simulink model "test_xeng_2"  (Simulink 7.0)
settings: Solver=ode45  StartTime=0.0  StopTime=200000  RelTol=1e-3
libraries: xbsIndex_r4 x1501, xbsReplacements_r4 x144, casper_library x23, xps_library x2, simulink x1
(part 2 of 16)

== system test_xeng_2/Subsystem/inj_vector1 ==
  In1 : Inport  OutDataType=sfix(16)  OutScaling=2^0
  Product : Product  OutDataType=sfix(16)  OutScaling=2^0  RndMeth=Zero
  err_clear_sim1 : Constant  Value=2^bit_pos  OutDataType=sfix(16)  OutScaling=2^0
  Out1 : Outport  OutDataType=sfix(16)  OutScaling=2^0
  wires:
  err_clear_sim1/1 -> Product/2
  In1/1 -> Product/1
  Product/1 -> Out1/1

== system test_xeng_2/Subsystem/new_acc2 ==
  In1 : Inport  OutDataType=sfix(16)  OutScaling=2^0
  Product : Product  OutDataType=sfix(16)  OutScaling=2^0  RndMeth=Zero
  err_clear_sim1 : Constant  Value=2^bit_pos  OutDataType=sfix(16)  OutScaling=2^0
  Out1 : Outport  OutDataType=sfix(16)  OutScaling=2^0
  wires:
  err_clear_sim1/1 -> Product/2
  In1/1 -> Product/1
  Product/1 -> Out1/1

== system test_xeng_2/Subsystem/run1 ==
  In1 : Inport  OutDataType=sfix(16)  OutScaling=2^0
  Product : Product  OutDataType=sfix(16)  OutScaling=2^0  RndMeth=Zero
  err_clear_sim1 : Constant  Value=2^bit_pos  OutDataType=sfix(16)  OutScaling=2^0
  Out1 : Outport  OutDataType=sfix(16)  OutScaling=2^0
  wires:
  err_clear_sim1/1 -> Product/2
  In1/1 -> Product/1
  Product/1 -> Out1/1

== system test_xeng_2/Subsystem/valid_sel1 ==
  In1 : Inport  OutDataType=sfix(16)  OutScaling=2^0
  Product : Product  OutDataType=sfix(16)  OutScaling=2^0  RndMeth=Zero
  err_clear_sim1 : Constant  Value=2^bit_pos  OutDataType=sfix(16)  OutScaling=2^0
  Out1 : Outport  OutDataType=sfix(16)  OutScaling=2^0
  wires:
  err_clear_sim1/1 -> Product/2
  In1/1 -> Product/1
  Product/1 -> Out1/1

== system test_xeng_2/pkt_reord0/deflagger ==
  din : Inport  OutDataType=sfix(16)  OutScaling=2^0
  Slice1 : xbsIndex_r4/Slice  nbits=16  boolean_output=off  mode=Lower Bit Location + Width  bit1=0  base1=MSB of Input  bit0=0  base0=LSB of Input  dbl_ovrd=off  block_type=slice
      settings: infoedit="Extracts a given range of bits from each input sample and presents it at the output.  The output type is ordinarily unsigned with binary point at zero, but can be Boolean when the slice is one bit wide.<P><P>Hardware notes: In hardware this block costs nothing."  block_version=10.1.3
  Slice2 : xbsIndex_r4/Slice  nbits=1  boolean_output=off  mode=Upper Bit Location + Width  bit1=-1  base1=MSB of Input  bit0=0  base0=LSB of Input  dbl_ovrd=off  block_type=slice
      settings: infoedit="Extracts a given range of bits from each input sample and presents it at the output.  The output type is ordinarily unsigned with binary point at zero, but can be Boolean when the slice is one bit wide.<P><P>Hardware notes: In hardware this block costs nothing."  block_version=10.1.3
  Slice3 : xbsIndex_r4/Slice  nbits=1  boolean_output=off  mode=Upper Bit Location + Width  bit1=0  base1=MSB of Input  bit0=0  base0=LSB of Input  dbl_ovrd=off  block_type=slice
      settings: infoedit="Extracts a given range of bits from each input sample and presents it at the output.  The output type is ordinarily unsigned with binary point at zero, but can be Boolean when the slice is one bit wide.<P><P>Hardware notes: In hardware this block costs nothing."  block_version=10.1.3
  dout : Outport  OutDataType=sfix(16)  OutScaling=2^0
  flag : Outport  Port=2  OutDataType=sfix(16)  OutScaling=2^0
  rcvd : Outport  Port=3  OutDataType=sfix(16)  OutScaling=2^0
  wires:
  Slice1/1 -> dout/1
  Slice3/1 -> rcvd/1
  Slice2/1 -> flag/1
  din/1 -> Slice3/1, Slice2/1, Slice1/1

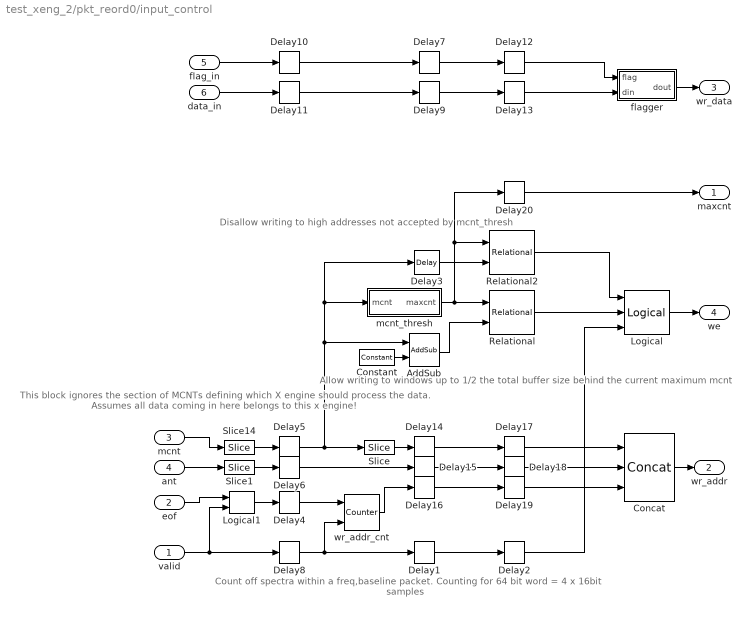
== system test_xeng_2/pkt_reord0/input_control ==
  note: Allow writing to windows
      | up to 1/2 the total buffer size
      |  behind the current maximum mcnt
  note: Count off spectra
      | within a freq,baseline
      | packet.  Counting for
      | 64 bit word = 4 x 16bit samples
  note: Disallow writing to high addresses
      | not accepted by mcnt_thresh
  note: This block ignores the section of
      | MCNTs defining which X engine
      | should process the data.
      | Assumes all data coming in here
      | belongs to this x engine!
  valid : Inport  OutDataType=sfix(16)  OutScaling=2^0
  eof : Inport  Port=2  OutDataType=sfix(16)  OutScaling=2^0
  mcnt : Inport  Port=3  OutDataType=sfix(16)  OutScaling=2^0
  ant : Inport  Port=4  OutDataType=sfix(16)  OutScaling=2^0
  flag_in : Inport  Port=5  OutDataType=sfix(16)  OutScaling=2^0
  data_in : Inport  Port=6  OutDataType=sfix(16)  OutScaling=2^0
  AddSub : xbsIndex_r4/AddSub  mode=Addition  use_carryin=off  use_carryout=off  en=off  latency=2  precision=User Defined  arith_type=Unsigned  n_bits=48 - ant_bits  bin_pt=0  quantization=Truncate  overflow=Wrap  dbl_ovrd=off  use_behavioral_HDL=on  pipelined=off  use_rpm=on  hw_selection=Fabric  block_type=addsub
      settings: xl_area=[0, 0, 0, 0, 0, 0, 0]  block_version=10.1.3
  Concat : xbsIndex_r4/Concat  num_inputs=3  dbl_ovrd=off  block_type=concat
      settings: block_version=10.1.3
  Constant : xbsIndex_r4/Constant  arith_type=Unsigned  const=2^(window_bits - 1)  n_bits=48 - ant_bits  bin_pt=0  explicit_period=on  period=1  equ=P=C  opselect=C  inp2=PCIN>>17  opr=+  inp1=P  carry=CIN  dbl_ovrd=off  block_type=constant
  Delay{1,7,9,14..16} (6 alike) : xbsIndex_r4/Delay  en=off  latency=2  dbl_ovrd=off  reg_retiming=on  block_type=delay
      settings: xl_area=[0, 0, 0, 0, 0, 0, 0]
  Delay{2,4..6,8,10..13,17..20} (13 alike) : xbsIndex_r4/Delay  en=off  latency=1  dbl_ovrd=off  reg_retiming=on  block_type=delay
      settings: xl_area=[0, 0, 0, 0, 0, 0, 0]
  Delay3 : xbsIndex_r4/Delay  en=off  latency=2  dbl_ovrd=off  reg_retiming=off  block_type=delay
      settings: xl_area=[0, 0, 0, 0, 0, 0, 0]
  Logical : xbsIndex_r4/Logical  logical_function=AND  inputs=3  en=off  latency=0  precision=Full  arith_type=Unsigned  n_bits=8  bin_pt=2  align_bp=on  dbl_ovrd=off  block_type=logical
      settings: xl_area=[0, 0, 0, 0, 0, 0, 0]
  Logical1 : xbsIndex_r4/Logical  logical_function=AND  inputs=2  en=off  latency=0  precision=Full  arith_type=Unsigned  n_bits=8  bin_pt=2  align_bp=on  dbl_ovrd=off  block_type=logical
      settings: xl_area=[0, 0, 0, 0, 0, 0, 0]
  Relational : xbsIndex_r4/Relational  mode=a<b  en=off  latency=1  dbl_ovrd=off  block_type=relational
      settings: xl_area=[0, 0, 0, 0, 0, 0, 0]  block_version=10.1.3
  Relational2 : xbsIndex_r4/Relational  mode=a>=b  en=off  latency=1  dbl_ovrd=off  block_type=relational
      settings: xl_area=[0, 0, 0, 0, 0, 0, 0]  block_version=10.1.3
  Slice : xbsIndex_r4/Slice  nbits=window_bits  boolean_output=off  mode=Lower Bit Location + Width  bit1=0  base1=MSB of Input  bit0=0  base0=LSB of Input  dbl_ovrd=off  block_type=slice
      settings: infoedit="Extracts a given range of bits from each input sample and presents it at the output.  The output type is ordinarily unsigned with binary point at zero, but can be Boolean when the slice is one bit wide.<P><P>Hardware notes: In hardware this block costs nothing."  block_version=10.1.3
  Slice1 : xbsIndex_r4/Slice  nbits=ant_bits  boolean_output=off  mode=Lower Bit Location + Width  bit1=0  base1=MSB of Input  bit0=0  base0=LSB of Input  dbl_ovrd=off  block_type=slice
      settings: infoedit="Extracts a given range of bits from each input sample and presents it at the output.  The output type is ordinarily unsigned with binary point at zero, but can be Boolean when the slice is one bit wide.<P><P>Hardware notes: In hardware this block costs nothing."  block_version=10.1.3
  Slice14 : xbsIndex_r4/Slice  nbits=ant_bits  boolean_output=off  mode=Two Bit Locations  bit1=0  base1=MSB of Input  bit0=xeng_bits  base0=LSB of Input  dbl_ovrd=off  block_type=slice
      settings: infoedit="Extracts a given range of bits from each input sample and presents it at the output.  The output type is ordinarily unsigned with binary point at zero, but can be Boolean when the slice is one bit wide.<P><P>Hardware notes: In hardware this block costs nothing."  block_version=10.1.3
  flagger : Subsystem
  mcnt_thresh : Subsystem
  wr_addr_cnt : xbsIndex_r4/Counter  cnt_type=Free Running  cnt_to=Inf  operation=Up  start_count=0  cnt_by_val=1  arith_type=Unsigned  n_bits=x_int_bits - 2  bin_pt=0  load_pin=off  rst=on  en=on  explicit_period=off  period=1  dbl_ovrd=off  use_behavioral_HDL=off  use_rpm=on  implementation=Fabric  block_type=counter
      settings: xl_area=[0, 0, 0, 0, 0, 0, 0]
  maxcnt : Outport  OutDataType=sfix(16)  OutScaling=2^0
  wr_addr : Outport  Port=2  OutDataType=sfix(16)  OutScaling=2^0
  wr_data : Outport  Port=3  OutDataType=sfix(16)  OutScaling=2^0
  we : Outport  Port=4  OutDataType=sfix(16)  OutScaling=2^0
  wires:
  Slice14/1 -> Delay5/1
  Delay3/1 -> Relational2/2
  Relational2/1 -> Logical/1
  mcnt_thresh/1(maxcnt) -> Relational2/1, Delay20/1, Relational/1
  Constant/1 -> AddSub/2
  AddSub/1 -> Relational/2
  Slice/1 -> Delay14/1
  Slice1/1 -> Delay6/1
  wr_addr_cnt/1 -> Delay16/1
  valid/1 -> Delay8/1, Logical1/2
  Relational/1 -> Logical/2
  Logical/1 -> we/1
  Delay2/1 -> Logical/3
  Delay4/1 -> wr_addr_cnt/1
  Delay8/1 -> wr_addr_cnt/2, Delay1/1
  mcnt/1 -> Slice14/1
  ant/1 -> Slice1/1
  Logical1/1 -> Delay4/1
  eof/1 -> Logical1/1
  Delay5/1 -> Delay3/1, mcnt_thresh/1(mcnt), AddSub/1, Slice/1
  Delay6/1 -> Delay15/1
  Delay7/1 -> Delay12/1
  data_in/1 -> Delay11/1
  Delay9/1 -> Delay13/1
  flag_in/1 -> Delay10/1
  flagger/1(dout) -> wr_data/1
  Delay10/1 -> Delay7/1
  Delay11/1 -> Delay9/1
  Delay12/1 -> flagger/1(flag)
  Delay13/1 -> flagger/2(din)
  Concat/1 -> wr_addr/1
  Delay1/1 -> Delay2/1
  Delay16/1 -> Delay19/1
  Delay15/1 -> Delay18/1
  Delay14/1 -> Delay17/1
  Delay17/1 -> Concat/1
  Delay18/1 -> Concat/2
  Delay19/1 -> Concat/3
  Delay20/1 -> maxcnt/1

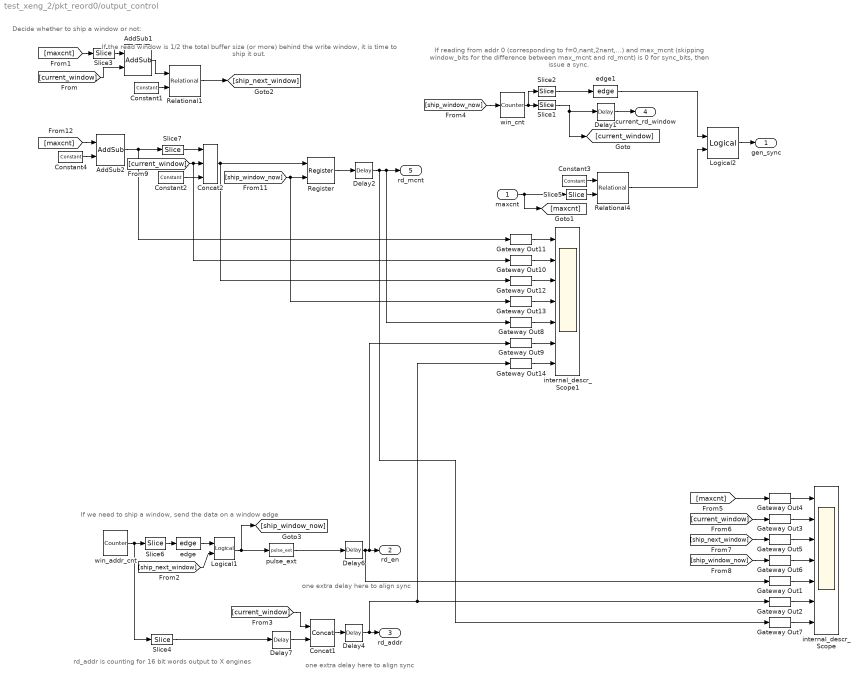
== system test_xeng_2/pkt_reord0/output_control ==
  note: one extra delay
      | here to align sync
  note: rd_addr is counting for
      | 16 bit words output to
      | X engines
  note: If the read window is 1/2
      | the total buffer size (or more)
      | behind the write window,
      | it is time to ship it out.
  note: one extra delay
      | here to align sync
  note: Decide whether to ship
      | a window or not:
  note: If we need to ship a window,
      | send the data on a window edge
  note: If reading from addr 0 (corresponding to f=0,nant,2nant,...)
      | and max_mcnt (skipping window_bits for the difference
      | between max_mcnt and rd_mcnt) is 0 for sync_bits, then
      | issue a sync.
  maxcnt : Inport  OutDataType=sfix(16)  OutScaling=2^0
  AddSub1 : xbsIndex_r4/AddSub  mode=Subtraction  use_carryin=off  use_carryout=off  en=off  latency=2  precision=User Defined  arith_type=Unsigned  n_bits=window_bits  bin_pt=0  quantization=Truncate  overflow=Wrap  dbl_ovrd=off  use_behavioral_HDL=on  pipelined=off  use_rpm=on  hw_selection=Fabric  block_type=addsub
      settings: xl_area=[0, 0, 0, 0, 0, 0, 0]  block_version=10.1.3
  AddSub2 : xbsIndex_r4/AddSub  mode=Subtraction  use_carryin=off  use_carryout=off  en=off  latency=2  precision=User Defined  arith_type=Unsigned  n_bits=48-xeng_bits  bin_pt=0  quantization=Truncate  overflow=Wrap  dbl_ovrd=off  use_behavioral_HDL=on  pipelined=off  use_rpm=on  hw_selection=Fabric  block_type=addsub
      settings: xl_area=[0, 0, 0, 0, 0, 0, 0]  block_version=10.1.3
  Concat1 : xbsIndex_r4/Concat  num_inputs=2  dbl_ovrd=off  block_type=concat
      settings: block_version=10.1.3
  Concat2 : xbsIndex_r4/Concat  num_inputs=3  dbl_ovrd=off  block_type=concat
      settings: block_version=10.1.3
  Constant1 : xbsIndex_r4/Constant  arith_type=Unsigned  const=2^(window_bits - 1)  n_bits=window_bits  bin_pt=0  explicit_period=on  period=1  equ=P=C  opselect=C  inp2=PCIN>>17  opr=+  inp1=P  carry=CIN  dbl_ovrd=off  block_type=constant
  Constant2 : xbsIndex_r4/Constant  arith_type=Unsigned  const=0  n_bits=xeng_bits  bin_pt=0  explicit_period=on  period=1  equ=P=C  opselect=C  inp2=PCIN>>17  opr=+  inp1=P  carry=CIN  dbl_ovrd=off  block_type=constant
  Constant3 : xbsIndex_r4/Constant  arith_type=Unsigned  const=0  n_bits=sync_bits - x_int_bits - ant_bits - window_bits  bin_pt=0  explicit_period=on  period=1  equ=P=C  opselect=C  inp2=PCIN>>17  opr=+  inp1=P  carry=CIN  dbl_ovrd=off  block_type=constant
  Constant4 : xbsIndex_r4/Constant  arith_type=Unsigned  const=2^(window_bits - 1)  n_bits=window_bits  bin_pt=0  explicit_period=on  period=1  equ=P=C  opselect=C  inp2=PCIN>>17  opr=+  inp1=P  carry=CIN  dbl_ovrd=off  block_type=constant
  Delay{1..2,4,6..7} (5 alike) : xbsIndex_r4/Delay  en=off  latency=1  dbl_ovrd=off  reg_retiming=off  block_type=delay
      settings: xl_area=[0, 0, 0, 0, 0, 0, 0]
  Gateway Out{1..14} (14 alike) : xbsIndex_r4/Gateway Out  hdl_port=off  timing_constraint=None  locs_specified=off  LOCs={}  block_type=gatewayout
      settings: infoedit="Gateway out block.  Converts Xilinx fixed point inputs into ouputs of type Simulink integer, double, or fixed point.<P><P>Hardware notes:  In hardware these blocks become top level output ports or are discarded, depending on how they are configured."  xl_area=[0, 0, 0, 0, 0, 0, 0]  block_version=10.1.3
  Logical1 : xbsIndex_r4/Logical  logical_function=AND  inputs=2  en=off  latency=0  precision=Full  arith_type=Unsigned  n_bits=8  bin_pt=2  align_bp=on  dbl_ovrd=off  block_type=logical
      settings: xl_area=[0, 0, 0, 0, 0, 0, 0]
  Logical2 : xbsIndex_r4/Logical  logical_function=AND  inputs=2  en=off  latency=0  precision=Full  arith_type=Unsigned  n_bits=8  bin_pt=2  align_bp=on  dbl_ovrd=off  block_type=logical
      settings: xl_area=[0, 0, 0, 0, 0, 0, 0]
  Register : xbsIndex_r4/Register  init=0  rst=off  en=on  dbl_ovrd=off  block_type=register
  Relational1 : xbsIndex_r4/Relational  mode=a>=b  en=off  latency=1  dbl_ovrd=off  block_type=relational
      settings: xl_area=[0, 0, 0, 0, 0, 0, 0]  block_version=10.1.3
  Relational4 : xbsIndex_r4/Relational  mode=a=b  en=off  latency=1  dbl_ovrd=off  block_type=relational
      settings: xl_area=[0, 0, 0, 0, 0, 0, 0]  block_version=10.1.3
  Slice1 : xbsIndex_r4/Slice  nbits=window_bits  boolean_output=off  mode=Lower Bit Location + Width  bit1=0  base1=MSB of Input  bit0=0  base0=LSB of Input  dbl_ovrd=off  block_type=slice
      settings: infoedit="Extracts a given range of bits from each input sample and presents it at the output.  The output type is ordinarily unsigned with binary point at zero, but can be Boolean when the slice is one bit wide.<P><P>Hardware notes: In hardware this block costs nothing."  block_version=10.1.3
  Slice2 : xbsIndex_r4/Slice  nbits=1  boolean_output=on  mode=Upper Bit Location + Width  bit1=0  base1=MSB of Input  bit0=0  base0=LSB of Input  dbl_ovrd=off  block_type=slice
      settings: infoedit="Extracts a given range of bits from each input sample and presents it at the output.  The output type is ordinarily unsigned with binary point at zero, but can be Boolean when the slice is one bit wide.<P><P>Hardware notes: In hardware this block costs nothing."  block_version=10.1.3
  Slice3 : xbsIndex_r4/Slice  nbits=window_bits  boolean_output=off  mode=Lower Bit Location + Width  bit1=0  base1=MSB of Input  bit0=0  base0=LSB of Input  dbl_ovrd=off  block_type=slice
      settings: infoedit="Extracts a given range of bits from each input sample and presents it at the output.  The output type is ordinarily unsigned with binary point at zero, but can be Boolean when the slice is one bit wide.<P><P>Hardware notes: In hardware this block costs nothing."  block_version=10.1.3
  Slice4 : xbsIndex_r4/Slice  nbits=x_int_bits + ant_bits  boolean_output=off  mode=Lower Bit Location + Width  bit1=0  base1=MSB of Input  bit0=0  base0=LSB of Input  dbl_ovrd=off  block_type=slice
      settings: infoedit="Extracts a given range of bits from each input sample and presents it at the output.  The output type is ordinarily unsigned with binary point at zero, but can be Boolean when the slice is one bit wide.<P><P>Hardware notes: In hardware this block costs nothing."  block_version=10.1.3
  Slice5 : xbsIndex_r4/Slice  nbits=window_bits  boolean_output=off  mode=Two Bit Locations  bit1=sync_bits - x_int_bits - ant_bits - 1  base1=LSB of Input  bit0=window_bits  base0=LSB of Input  dbl_ovrd=off  block_type=slice
      settings: infoedit="Extracts a given range of bits from each input sample and presents it at the output.  The output type is ordinarily unsigned with binary point at zero, but can be Boolean when the slice is one bit wide.<P><P>Hardware notes: In hardware this block costs nothing."  block_version=10.1.3
  Slice6 : xbsIndex_r4/Slice  nbits=1  boolean_output=on  mode=Upper Bit Location + Width  bit1=0  base1=MSB of Input  bit0=0  base0=LSB of Input  dbl_ovrd=off  block_type=slice
      settings: infoedit="Extracts a given range of bits from each input sample and presents it at the output.  The output type is ordinarily unsigned with binary point at zero, but can be Boolean when the slice is one bit wide.<P><P>Hardware notes: In hardware this block costs nothing."  block_version=10.1.3
  Slice7 : xbsIndex_r4/Slice  nbits=1  boolean_output=off  mode=Two Bit Locations  bit1=0  base1=MSB of Input  bit0=window_bits  base0=LSB of Input  dbl_ovrd=off  block_type=slice
      settings: infoedit="Extracts a given range of bits from each input sample and presents it at the output.  The output type is ordinarily unsigned with binary point at zero, but can be Boolean when the slice is one bit wide.<P><P>Hardware notes: In hardware this block costs nothing."  block_version=10.1.3
  edge : casper_library/Misc/edge  SystemSampleTime=-1
  edge1 : casper_library/Misc/edge  SystemSampleTime=-1
  internal_descr_Scope : Scope  NumInputPorts=7
      settings: TimeRange=1  YMin=-1~-1~0.95~-5~-5~-5~-5  YMax=1~1~1.05~5~5~5~5  SaveName=ScopeData2
  internal_descr_Scope1 : Scope  NumInputPorts=7
      settings: TimeRange=1  YMin=-1~-1~0.95~-5~-5~-5~-5  YMax=1~1~1.05~5~5~5~5  SaveName=ScopeData4
  pulse_ext : casper_library/Misc/pulse_ext  SystemSampleTime=-1  pulse_len=2^(x_int_bits + ant_bits)
  win_addr_cnt : xbsIndex_r4/Counter  cnt_type=Free Running  cnt_to=Inf  operation=Up  start_count=0  cnt_by_val=1  arith_type=Unsigned  n_bits=x_int_bits + ant_bits + 1  bin_pt=0  load_pin=off  rst=off  en=off  explicit_period=off  period=1  dbl_ovrd=off  use_behavioral_HDL=off  use_rpm=on  implementation=Fabric  block_type=counter
      settings: xl_area=[0, 0, 0, 0, 0, 0, 0]
  win_cnt : xbsIndex_r4/Counter  cnt_type=Free Running  cnt_to=Inf  operation=Up  start_count=0  cnt_by_val=1  arith_type=Unsigned  n_bits=window_bits + 1  bin_pt=0  load_pin=off  rst=off  en=on  explicit_period=off  period=1  dbl_ovrd=off  use_behavioral_HDL=off  use_rpm=on  implementation=Fabric  block_type=counter
      settings: xl_area=[0, 0, 0, 0, 0, 0, 0]
  gen_sync : Outport  OutDataType=sfix(16)  OutScaling=2^0
  rd_en : Outport  Port=2  OutDataType=sfix(16)  OutScaling=2^0
  rd_addr : Outport  Port=3  OutDataType=sfix(16)  OutScaling=2^0
  current_rd_window : Outport  Port=4  OutDataType=sfix(16)  OutScaling=2^0
  rd_mcnt : Outport  Port=5  OutDataType=sfix(16)  OutScaling=2^0
  wires:
  pulse_ext/1 -> Delay6/1
  Concat1/1 -> Delay4/1
  Delay7/1 -> Concat1/2
  Slice2/1 -> edge1/1
  Slice1/1 -> [current_window], Delay1/1
  Slice4/1 -> Delay7/1
  edge/1 -> Logical1/1
  Slice6/1 -> edge/1
  win_addr_cnt/1 -> Slice4/1, Slice6/1
  Slice5/1 -> Relational4/2
  Constant3/1 -> Relational4/1
  edge1/1 -> Logical2/1
  Logical1/1 -> pulse_ext/1, [ship_window_now]
  win_cnt/1 -> Slice2/1, Slice1/1
  maxcnt/1 -> Slice5/1, [maxcnt]
  Logical2/1 -> gen_sync/1
  Delay6/1 -> Gateway Out1/1, rd_en/1, Gateway Out9/1
  [ship_next_window] -> Logical1/2
  Delay4/1 -> rd_addr/1, Gateway Out2/1, Gateway Out14/1
  Slice3/1 -> AddSub1/1
  AddSub1/1 -> Relational1/1
  Constant1/1 -> Relational1/2
  [current_window] -> AddSub1/2
  [maxcnt] -> Slice3/1
  Relational1/1 -> [ship_next_window]
  [ship_window_now] -> win_cnt/1
  Relational4/1 -> Logical2/2
  Gateway Out3/1 -> internal_descr_Scope/2
  Gateway Out4/1 -> internal_descr_Scope/1
  Gateway Out5/1 -> internal_descr_Scope/3
  [maxcnt] -> Gateway Out4/1
  [current_window] -> Gateway Out3/1
  [ship_next_window] -> Gateway Out5/1
  [current_window] -> Concat1/1
  Gateway Out6/1 -> internal_descr_Scope/4
  Gateway Out1/1 -> internal_descr_Scope/5
  Gateway Out2/1 -> internal_descr_Scope/6
  [ship_window_now] -> Gateway Out6/1
  Delay1/1 -> current_rd_window/1
  AddSub2/1 -> Slice7/1, Gateway Out11/1
  Slice7/1 -> Concat2/1
  Concat2/1 -> Register/1, Gateway Out12/1
  [ship_window_now] -> Register/2, Gateway Out13/1
  Gateway Out7/1 -> internal_descr_Scope/7
  Constant2/1 -> Concat2/3
  [current_window] -> Concat2/2, Gateway Out10/1
  Register/1 -> Delay2/1
  Constant4/1 -> AddSub2/2
  [maxcnt] -> AddSub2/1
  Gateway Out10/1 -> internal_descr_Scope1/2
  Gateway Out11/1 -> internal_descr_Scope1/1
  Gateway Out12/1 -> internal_descr_Scope1/3
  Gateway Out13/1 -> internal_descr_Scope1/4
  Gateway Out8/1 -> internal_descr_Scope1/5
  Gateway Out9/1 -> internal_descr_Scope1/6
  Gateway Out14/1 -> internal_descr_Scope1/7
  Delay2/1 -> Gateway Out7/1, rd_mcnt/1, Gateway Out8/1

== system test_xeng_2/xeng/baseline_tap2 ==
  a_del : Inport  OutDataType=sfix(16)  OutScaling=2^0
  a_ndel : Inport  Port=2  OutDataType=sfix(16)  OutScaling=2^0
  a_end : Inport  Port=3  OutDataType=sfix(16)  OutScaling=2^0
  acc_in : Inport  Port=4  OutDataType=sfix(16)  OutScaling=2^0
  valid_in : Inport  Port=5  OutDataType=sfix(16)  OutScaling=2^0
  rst : Inport  Port=6  OutDataType=sfix(16)  OutScaling=2^0
  sync1 : Inport  Port=7  OutDataType=sfix(16)  OutScaling=2^0
  Constant : xbsIndex_r4/Constant  arith_type=Unsigned  const=ant_sep * acc_len  n_bits=ant_bits + bit_growth  bin_pt=0  explicit_period=off  period=1  equ=P=C  opselect=C  inp2=PCIN>>17  opr=+  inp1=P  carry=CIN  dbl_ovrd=off  block_type=constant
      settings: block_version=9.1.01
  Convert : xbsIndex_r4/Convert  arith_type=Unsigned  n_bits=1  bin_pt=0  quantization=Truncate  overflow=Wrap  latency=0  dbl_ovrd=off  pipeline=off  block_type=convert
      settings: xl_area=[0, 0, 0, 0, 0, 0, 0]
  Counter : xbsIndex_r4/Counter  cnt_type=Count Limited  cnt_to=n_ants * acc_len - 1  operation=Up  start_count=0  cnt_by_val=1  arith_type=Unsigned  n_bits=ant_bits + bit_growth  bin_pt=0  load_pin=off  rst=on  en=off  explicit_period=off  period=1  dbl_ovrd=off  use_behavioral_HDL=off  use_rpm=on  implementation=Fabric  block_type=counter
      settings: xl_area=[0, 0, 0, 0, 0, 0, 0]  block_version=9.1.01
  Delay{1,3,7..8} (4 alike) : xbsIndex_r4/Delay  en=off  latency=1  dbl_ovrd=off  reg_retiming=off  block_type=delay
      settings: xl_area=[0, 0, 0, 0, 0, 0, 0]  block_version=9.1.01
  Mux : xbsIndex_r4/Mux  inputs=2  en=off  latency=1  precision=Full  arith_type="Signed  (2's comp)"  n_bits=8  bin_pt=2  quantization=Truncate  overflow=Wrap  dbl_ovrd=off  block_type=mux
      settings: xl_area=[0, 0, 0, 0, 0, 0, 0]  block_version=9.1.01
  Relational : xbsIndex_r4/Relational  mode=a<b  en=off  latency=0  dbl_ovrd=off  block_type=relational
      settings: xl_area=[0, 0, 0, 0, 0, 0, 0]  block_version=9.1.01
  delay : Subsystem  AncestorBlock=casper_library/Delays/delay_bram  mask(delay_bram){DelayLen=acc_len, bram_latency=bram_latency}
      mask prompts: DelayLen "Delay By:"; bram_latency "BRAM Latency"
      mask help: A delay block that uses BRAM for its storage.
      mask init:
      | if (DelayLen <= bram_latency)
      | 	error('delay value must be greater than BRAM Latency');
      | end
      | BitWidth = max(ceil(log2(DelayLen)), 2);
      mask Help: eval('xlWeb([getenv(''MLIB_ROOT''), ''\doc\html\sp_delay_bram\sp_delay_bram.html''])')
  dual_pol_cmac : Subsystem
  a_del_out : Outport  OutDataType=sfix(16)  OutScaling=2^0
  a_ndel_out : Outport  Port=2  OutDataType=sfix(16)  OutScaling=2^0
  a_end_out : Outport  Port=3  OutDataType=sfix(16)  OutScaling=2^0
  acc_out : Outport  Port=4  OutDataType=sfix(16)  OutScaling=2^0
  valid_out : Outport  Port=5  OutDataType=sfix(16)  OutScaling=2^0
  rst_out : Outport  Port=6  OutDataType=sfix(16)  OutScaling=2^0
  sync_out : Outport  Port=7  OutDataType=sfix(16)  OutScaling=2^0
  wires:
  delay/1(Out1) -> Delay3/1
  Mux/1 -> dual_pol_cmac/2(a2)
  Counter/1 -> Relational/1
  Constant/1 -> Relational/2
  Relational/1 -> Convert/1
  Convert/1 -> Mux/1
  rst/1 -> Delay1/1, Counter/1
  a_del/1 -> delay/1(In1)
  dual_pol_cmac/1(acc_out) -> acc_out/1
  acc_in/1 -> dual_pol_cmac/3(acc_in)
  dual_pol_cmac/2(valid_out) -> valid_out/1
  valid_in/1 -> dual_pol_cmac/5(valid_in)
  a_ndel/1 -> Mux/2, Delay7/1
  a_end/1 -> Mux/3, Delay8/1
  Delay3/1 -> dual_pol_cmac/1(a1), a_del_out/1
  Delay7/1 -> a_ndel_out/1
  Delay8/1 -> a_end_out/1
  Delay1/1 -> dual_pol_cmac/4(sync), rst_out/1
  sync1/1 -> sync_out/1

== system test_xeng_2/xeng/baseline_tap3 ==
  a_del : Inport  OutDataType=sfix(16)  OutScaling=2^0
  a_ndel : Inport  Port=2  OutDataType=sfix(16)  OutScaling=2^0
  a_end : Inport  Port=3  OutDataType=sfix(16)  OutScaling=2^0
  acc_in : Inport  Port=4  OutDataType=sfix(16)  OutScaling=2^0
  valid_in : Inport  Port=5  OutDataType=sfix(16)  OutScaling=2^0
  rst : Inport  Port=6  OutDataType=sfix(16)  OutScaling=2^0
  sync1 : Inport  Port=7  OutDataType=sfix(16)  OutScaling=2^0
  Constant : xbsIndex_r4/Constant  arith_type=Unsigned  const=ant_sep * acc_len  n_bits=ant_bits + bit_growth  bin_pt=0  explicit_period=off  period=1  equ=P=C  opselect=C  inp2=PCIN>>17  opr=+  inp1=P  carry=CIN  dbl_ovrd=off  block_type=constant
      settings: block_version=9.1.01
  Convert : xbsIndex_r4/Convert  arith_type=Unsigned  n_bits=1  bin_pt=0  quantization=Truncate  overflow=Wrap  latency=0  dbl_ovrd=off  pipeline=off  block_type=convert
      settings: xl_area=[0, 0, 0, 0, 0, 0, 0]
  Counter : xbsIndex_r4/Counter  cnt_type=Count Limited  cnt_to=n_ants * acc_len - 1  operation=Up  start_count=0  cnt_by_val=1  arith_type=Unsigned  n_bits=ant_bits + bit_growth  bin_pt=0  load_pin=off  rst=on  en=off  explicit_period=off  period=1  dbl_ovrd=off  use_behavioral_HDL=off  use_rpm=on  implementation=Fabric  block_type=counter
      settings: xl_area=[0, 0, 0, 0, 0, 0, 0]  block_version=9.1.01
  Delay{1,3,7..8} (4 alike) : xbsIndex_r4/Delay  en=off  latency=1  dbl_ovrd=off  reg_retiming=off  block_type=delay
      settings: xl_area=[0, 0, 0, 0, 0, 0, 0]  block_version=9.1.01
  Mux : xbsIndex_r4/Mux  inputs=2  en=off  latency=1  precision=Full  arith_type="Signed  (2's comp)"  n_bits=8  bin_pt=2  quantization=Truncate  overflow=Wrap  dbl_ovrd=off  block_type=mux
      settings: xl_area=[0, 0, 0, 0, 0, 0, 0]  block_version=9.1.01
  Relational : xbsIndex_r4/Relational  mode=a<b  en=off  latency=0  dbl_ovrd=off  block_type=relational
      settings: xl_area=[0, 0, 0, 0, 0, 0, 0]  block_version=9.1.01
  delay : Subsystem  AncestorBlock=casper_library/Delays/delay_bram  mask(delay_bram){DelayLen=acc_len, bram_latency=bram_latency}
      mask prompts: DelayLen "Delay By:"; bram_latency "BRAM Latency"
      mask help: A delay block that uses BRAM for its storage.
      mask init:
      | if (DelayLen <= bram_latency)
      | 	error('delay value must be greater than BRAM Latency');
      | end
      | BitWidth = max(ceil(log2(DelayLen)), 2);
      mask Help: eval('xlWeb([getenv(''MLIB_ROOT''), ''\doc\html\sp_delay_bram\sp_delay_bram.html''])')
  dual_pol_cmac : Subsystem
  a_del_out : Outport  OutDataType=sfix(16)  OutScaling=2^0
  a_ndel_out : Outport  Port=2  OutDataType=sfix(16)  OutScaling=2^0
  a_end_out : Outport  Port=3  OutDataType=sfix(16)  OutScaling=2^0
  acc_out : Outport  Port=4  OutDataType=sfix(16)  OutScaling=2^0
  valid_out : Outport  Port=5  OutDataType=sfix(16)  OutScaling=2^0
  rst_out : Outport  Port=6  OutDataType=sfix(16)  OutScaling=2^0
  sync_out : Outport  Port=7  OutDataType=sfix(16)  OutScaling=2^0
  wires:
  delay/1(Out1) -> Delay3/1
  Mux/1 -> dual_pol_cmac/2(a2)
  Counter/1 -> Relational/1
  Constant/1 -> Relational/2
  Relational/1 -> Convert/1
  Convert/1 -> Mux/1
  rst/1 -> Delay1/1, Counter/1
  a_del/1 -> delay/1(In1)
  dual_pol_cmac/1(acc_out) -> acc_out/1
  acc_in/1 -> dual_pol_cmac/3(acc_in)
  dual_pol_cmac/2(valid_out) -> valid_out/1
  valid_in/1 -> dual_pol_cmac/5(valid_in)
  a_ndel/1 -> Mux/2, Delay7/1
  a_end/1 -> Mux/3, Delay8/1
  Delay3/1 -> dual_pol_cmac/1(a1), a_del_out/1
  Delay7/1 -> a_ndel_out/1
  Delay8/1 -> a_end_out/1
  Delay1/1 -> dual_pol_cmac/4(sync), rst_out/1
  sync1/1 -> sync_out/1

== system test_xeng_2/xeng/baseline_tap4 ==
  a_del : Inport  OutDataType=sfix(16)  OutScaling=2^0
  a_ndel : Inport  Port=2  OutDataType=sfix(16)  OutScaling=2^0
  a_end : Inport  Port=3  OutDataType=sfix(16)  OutScaling=2^0
  acc_in : Inport  Port=4  OutDataType=sfix(16)  OutScaling=2^0
  valid_in : Inport  Port=5  OutDataType=sfix(16)  OutScaling=2^0
  rst : Inport  Port=6  OutDataType=sfix(16)  OutScaling=2^0
  sync1 : Inport  Port=7  OutDataType=sfix(16)  OutScaling=2^0
  Constant : xbsIndex_r4/Constant  arith_type=Unsigned  const=ant_sep * acc_len  n_bits=ant_bits + bit_growth  bin_pt=0  explicit_period=off  period=1  equ=P=C  opselect=C  inp2=PCIN>>17  opr=+  inp1=P  carry=CIN  dbl_ovrd=off  block_type=constant
      settings: block_version=9.1.01
  Convert : xbsIndex_r4/Convert  arith_type=Unsigned  n_bits=1  bin_pt=0  quantization=Truncate  overflow=Wrap  latency=0  dbl_ovrd=off  pipeline=off  block_type=convert
      settings: xl_area=[0, 0, 0, 0, 0, 0, 0]
  Counter : xbsIndex_r4/Counter  cnt_type=Count Limited  cnt_to=n_ants * acc_len - 1  operation=Up  start_count=0  cnt_by_val=1  arith_type=Unsigned  n_bits=ant_bits + bit_growth  bin_pt=0  load_pin=off  rst=on  en=off  explicit_period=off  period=1  dbl_ovrd=off  use_behavioral_HDL=off  use_rpm=on  implementation=Fabric  block_type=counter
      settings: xl_area=[0, 0, 0, 0, 0, 0, 0]  block_version=9.1.01
  Delay{1,3,7..8} (4 alike) : xbsIndex_r4/Delay  en=off  latency=1  dbl_ovrd=off  reg_retiming=off  block_type=delay
      settings: xl_area=[0, 0, 0, 0, 0, 0, 0]  block_version=9.1.01
  Mux : xbsIndex_r4/Mux  inputs=2  en=off  latency=1  precision=Full  arith_type="Signed  (2's comp)"  n_bits=8  bin_pt=2  quantization=Truncate  overflow=Wrap  dbl_ovrd=off  block_type=mux
      settings: xl_area=[0, 0, 0, 0, 0, 0, 0]  block_version=9.1.01
  Relational : xbsIndex_r4/Relational  mode=a<b  en=off  latency=0  dbl_ovrd=off  block_type=relational
      settings: xl_area=[0, 0, 0, 0, 0, 0, 0]  block_version=9.1.01
  delay : Subsystem  AncestorBlock=casper_library/Delays/delay_bram  mask(delay_bram){DelayLen=acc_len, bram_latency=bram_latency}
      mask prompts: DelayLen "Delay By:"; bram_latency "BRAM Latency"
      mask help: A delay block that uses BRAM for its storage.
      mask init:
      | if (DelayLen <= bram_latency)
      | 	error('delay value must be greater than BRAM Latency');
      | end
      | BitWidth = max(ceil(log2(DelayLen)), 2);
      mask Help: eval('xlWeb([getenv(''MLIB_ROOT''), ''\doc\html\sp_delay_bram\sp_delay_bram.html''])')
  dual_pol_cmac : Subsystem
  a_del_out : Outport  OutDataType=sfix(16)  OutScaling=2^0
  a_ndel_out : Outport  Port=2  OutDataType=sfix(16)  OutScaling=2^0
  a_end_out : Outport  Port=3  OutDataType=sfix(16)  OutScaling=2^0
  acc_out : Outport  Port=4  OutDataType=sfix(16)  OutScaling=2^0
  valid_out : Outport  Port=5  OutDataType=sfix(16)  OutScaling=2^0
  rst_out : Outport  Port=6  OutDataType=sfix(16)  OutScaling=2^0
  sync_out : Outport  Port=7  OutDataType=sfix(16)  OutScaling=2^0
  wires:
  delay/1(Out1) -> Delay3/1
  Mux/1 -> dual_pol_cmac/2(a2)
  Counter/1 -> Relational/1
  Constant/1 -> Relational/2
  Relational/1 -> Convert/1
  Convert/1 -> Mux/1
  rst/1 -> Delay1/1, Counter/1
  a_del/1 -> delay/1(In1)
  dual_pol_cmac/1(acc_out) -> acc_out/1
  acc_in/1 -> dual_pol_cmac/3(acc_in)
  dual_pol_cmac/2(valid_out) -> valid_out/1
  valid_in/1 -> dual_pol_cmac/5(valid_in)
  a_ndel/1 -> Mux/2, Delay7/1
  a_end/1 -> Mux/3, Delay8/1
  Delay3/1 -> dual_pol_cmac/1(a1), a_del_out/1
  Delay7/1 -> a_ndel_out/1
  Delay8/1 -> a_end_out/1
  Delay1/1 -> dual_pol_cmac/4(sync), rst_out/1
  sync1/1 -> sync_out/1

== system test_xeng_2/xeng/xeng_conj_fix ==
  acc : Inport  OutDataType=sfix(16)  OutScaling=2^0
  valid : Inport  Port=2  OutDataType=sfix(16)  OutScaling=2^0
  sync : Inport  Port=3  OutDataType=sfix(16)  OutScaling=2^0
  delay{1..5} (5 alike) : xbsIndex_r4/Delay  en=off  latency=1  dbl_ovrd=off  reg_retiming=on  block_type=delay
  imag_sel : xbsIndex_r4/Mux  inputs=2  en=off  latency=1  precision=Full  arith_type=Unsigned  n_bits=16  bin_pt=14  quantization=Truncate  overflow=Wrap  dbl_ovrd=off  block_type=mux
      settings: AttributesFormatString=num_ants=8
  negate : xbsIndex_r4/Negate  precision=User Defined  arith_type="Signed  (2's comp)"  n_bits=4  bin_pt=0  quantization=Truncate  overflow=Wrap  en=off  latency=0  dbl_ovrd=off  block_type=negate
      settings: block_version=10.1.3
  pivot : xbsIndex_r4/Relational  mode=a>=b  en=off  latency=1  dbl_ovrd=off  block_type=relational
      settings: block_version=10.1.3
  pivot_point : xbsIndex_r4/Constant  arith_type=Unsigned  const=240  n_bits=9  bin_pt=0  explicit_period=off  period=1  equ=P=C  opselect=C  inp2=PCIN>>17  opr=+  inp1=P  carry=CIN  dbl_ovrd=off  block_type=constant
  pos_cnt : xbsIndex_r4/Counter  cnt_type=Count Limited  cnt_to=287  operation=Up  start_count=0  cnt_by_val=1  arith_type=Unsigned  n_bits=9  bin_pt=0  load_pin=off  rst=on  en=on  explicit_period=on  period=1  dbl_ovrd=off  use_behavioral_HDL=off  use_rpm=off  implementation=Fabric  block_type=counter
  reint_in : xbsIndex_r4/Reinterpret  force_arith_type=on  arith_type="Signed  (2's comp)"  force_bin_pt=on  bin_pt=0  block_type=reinterpret
      settings: infoedit="Changes signal type without altering the binary representation.   You can changed the signal between signed and unsigned, and relocate the binary point.<P><P>Hardware notes: In hardware this block costs nothing.<P><P>Example:  Suppose the input is 6 bits wide, signed, with 2 fractional bits, and the output is forced to unsigned with 0 fractional bits.  Then an input of -2.0 (1110.00 in binary 2's complement) becomes an output of 56 (111000 in binary)."  block_version=10.1.3
  reint_out : xbsIndex_r4/Reinterpret  force_arith_type=on  arith_type=Unsigned  force_bin_pt=on  bin_pt=0  block_type=reinterpret
      settings: infoedit="Changes signal type without altering the binary representation.   You can changed the signal between signed and unsigned, and relocate the binary point.<P><P>Hardware notes: In hardware this block costs nothing.<P><P>Example:  Suppose the input is 6 bits wide, signed, with 2 fractional bits, and the output is forced to unsigned with 0 fractional bits.  Then an input of -2.0 (1110.00 in binary 2's complement) becomes an output of 56 (111000 in binary)."  block_version=10.1.3
  sel_conj : xbsIndex_r4/Mux  inputs=2  en=off  latency=1  precision=Full  arith_type=Unsigned  n_bits=16  bin_pt=14  quantization=Truncate  overflow=Wrap  dbl_ovrd=off  block_type=mux
  slice : xbsIndex_r4/Slice  nbits=1  boolean_output=off  mode=Lower Bit Location + Width  bit1=0  base1=MSB of Input  bit0=0  base0=LSB of Input  dbl_ovrd=off  block_type=slice
      settings: infoedit="Extracts a given range of bits from each input sample and presents it at the output.  The output type is ordinarily unsigned with binary point at zero, but can be Boolean when the slice is one bit wide.<P><P>Hardware notes: In hardware this block costs nothing."  block_version=10.1.3
  acc_out : Outport
  valid_out : Outport  Port=2
  sync_out : Outport  Port=3
  wires:
  acc/1 -> delay1/1
  valid/1 -> delay2/1, pos_cnt/1
  sync/1 -> delay3/1, pos_cnt/2
  delay2/1 -> delay4/1
  delay3/1 -> delay5/1
  delay4/1 -> valid_out/1
  delay5/1 -> sync_out/1
  pos_cnt/1 -> pivot/1, slice/1
  pivot_point/1 -> pivot/2
  pivot/1 -> sel_conj/1
  delay1/1 -> sel_conj/2, reint_in/1, imag_sel/2
  sel_conj/1 -> acc_out/1
  reint_in/1 -> negate/1
  slice/1 -> imag_sel/1
  negate/1 -> reint_out/1
  reint_out/1 -> imag_sel/3
  imag_sel/1 -> sel_conj/3

== system test_xeng_2/xeng_static/baseline_tap2 ==
  a_del : Inport  OutDataType=sfix(16)  OutScaling=2^0
  a_ndel : Inport  Port=2  OutDataType=sfix(16)  OutScaling=2^0
  a_end : Inport  Port=3  OutDataType=sfix(16)  OutScaling=2^0
  acc_in : Inport  Port=4  OutDataType=sfix(16)  OutScaling=2^0
  valid_in : Inport  Port=5  OutDataType=sfix(16)  OutScaling=2^0
  rst : Inport  Port=6  OutDataType=sfix(16)  OutScaling=2^0
  sync1 : Inport  Port=7  OutDataType=sfix(16)  OutScaling=2^0
  Constant : xbsIndex_r4/Constant  arith_type=Unsigned  const=ant_sep * acc_len  n_bits=ant_bits + bit_growth  bin_pt=0  explicit_period=off  period=1  equ=P=C  opselect=C  inp2=PCIN>>17  opr=+  inp1=P  carry=CIN  dbl_ovrd=off  block_type=constant
      settings: block_version=9.1.01
  Convert : xbsIndex_r4/Convert  arith_type=Unsigned  n_bits=1  bin_pt=0  quantization=Truncate  overflow=Wrap  latency=0  dbl_ovrd=off  pipeline=off  block_type=convert
      settings: xl_area=[0, 0, 0, 0, 0, 0, 0]
  Counter : xbsIndex_r4/Counter  cnt_type=Count Limited  cnt_to=n_ants * acc_len - 1  operation=Up  start_count=0  cnt_by_val=1  arith_type=Unsigned  n_bits=ant_bits + bit_growth  bin_pt=0  load_pin=off  rst=on  en=off  explicit_period=off  period=1  dbl_ovrd=off  use_behavioral_HDL=off  use_rpm=on  implementation=Fabric  block_type=counter
      settings: xl_area=[0, 0, 0, 0, 0, 0, 0]  block_version=9.1.01
  Delay{1,3,7..8} (4 alike) : xbsIndex_r4/Delay  en=off  latency=1  dbl_ovrd=off  reg_retiming=off  block_type=delay
      settings: xl_area=[0, 0, 0, 0, 0, 0, 0]  block_version=9.1.01
  Mux : xbsIndex_r4/Mux  inputs=2  en=off  latency=1  precision=Full  arith_type="Signed  (2's comp)"  n_bits=8  bin_pt=2  quantization=Truncate  overflow=Wrap  dbl_ovrd=off  block_type=mux
      settings: xl_area=[0, 0, 0, 0, 0, 0, 0]  block_version=9.1.01
  Relational : xbsIndex_r4/Relational  mode=a<b  en=off  latency=0  dbl_ovrd=off  block_type=relational
      settings: xl_area=[0, 0, 0, 0, 0, 0, 0]  block_version=9.1.01
  delay : Subsystem  AncestorBlock=casper_library/Delays/delay_bram  mask(delay_bram){DelayLen=acc_len, bram_latency=bram_latency}
      mask prompts: DelayLen "Delay By:"; bram_latency "BRAM Latency"
      mask help: A delay block that uses BRAM for its storage.
      mask init:
      | if (DelayLen <= bram_latency)
      | 	error('delay value must be greater than BRAM Latency');
      | end
      | BitWidth = max(ceil(log2(DelayLen)), 2);
      mask Help: eval('xlWeb([getenv(''MLIB_ROOT''), ''\doc\html\sp_delay_bram\sp_delay_bram.html''])')
  dual_pol_cmac : Subsystem
  a_del_out : Outport  OutDataType=sfix(16)  OutScaling=2^0
  a_ndel_out : Outport  Port=2  OutDataType=sfix(16)  OutScaling=2^0
  a_end_out : Outport  Port=3  OutDataType=sfix(16)  OutScaling=2^0
  acc_out : Outport  Port=4  OutDataType=sfix(16)  OutScaling=2^0
  valid_out : Outport  Port=5  OutDataType=sfix(16)  OutScaling=2^0
  rst_out : Outport  Port=6  OutDataType=sfix(16)  OutScaling=2^0
  sync_out : Outport  Port=7  OutDataType=sfix(16)  OutScaling=2^0
  wires:
  delay/1(Out1) -> Delay3/1
  Mux/1 -> dual_pol_cmac/2(a2)
  Counter/1 -> Relational/1
  Constant/1 -> Relational/2
  Relational/1 -> Convert/1
  Convert/1 -> Mux/1
  rst/1 -> Delay1/1, Counter/1
  a_del/1 -> delay/1(In1)
  dual_pol_cmac/1(acc_out) -> acc_out/1
  acc_in/1 -> dual_pol_cmac/3(acc_in)
  dual_pol_cmac/2(valid_out) -> valid_out/1
  valid_in/1 -> dual_pol_cmac/5(valid_in)
  a_ndel/1 -> Mux/2, Delay7/1
  a_end/1 -> Mux/3, Delay8/1
  Delay3/1 -> dual_pol_cmac/1(a1), a_del_out/1
  Delay7/1 -> a_ndel_out/1
  Delay8/1 -> a_end_out/1
  Delay1/1 -> dual_pol_cmac/4(sync), rst_out/1
  sync1/1 -> sync_out/1

== system test_xeng_2/xeng_static/baseline_tap3 ==
  a_del : Inport  OutDataType=sfix(16)  OutScaling=2^0
  a_ndel : Inport  Port=2  OutDataType=sfix(16)  OutScaling=2^0
  a_end : Inport  Port=3  OutDataType=sfix(16)  OutScaling=2^0
  acc_in : Inport  Port=4  OutDataType=sfix(16)  OutScaling=2^0
  valid_in : Inport  Port=5  OutDataType=sfix(16)  OutScaling=2^0
  rst : Inport  Port=6  OutDataType=sfix(16)  OutScaling=2^0
  sync1 : Inport  Port=7  OutDataType=sfix(16)  OutScaling=2^0
  Constant : xbsIndex_r4/Constant  arith_type=Unsigned  const=ant_sep * acc_len  n_bits=ant_bits + bit_growth  bin_pt=0  explicit_period=off  period=1  equ=P=C  opselect=C  inp2=PCIN>>17  opr=+  inp1=P  carry=CIN  dbl_ovrd=off  block_type=constant
      settings: block_version=9.1.01
  Convert : xbsIndex_r4/Convert  arith_type=Unsigned  n_bits=1  bin_pt=0  quantization=Truncate  overflow=Wrap  latency=0  dbl_ovrd=off  pipeline=off  block_type=convert
      settings: xl_area=[0, 0, 0, 0, 0, 0, 0]
  Counter : xbsIndex_r4/Counter  cnt_type=Count Limited  cnt_to=n_ants * acc_len - 1  operation=Up  start_count=0  cnt_by_val=1  arith_type=Unsigned  n_bits=ant_bits + bit_growth  bin_pt=0  load_pin=off  rst=on  en=off  explicit_period=off  period=1  dbl_ovrd=off  use_behavioral_HDL=off  use_rpm=on  implementation=Fabric  block_type=counter
      settings: xl_area=[0, 0, 0, 0, 0, 0, 0]  block_version=9.1.01
  Delay{1,3,7..8} (4 alike) : xbsIndex_r4/Delay  en=off  latency=1  dbl_ovrd=off  reg_retiming=off  block_type=delay
      settings: xl_area=[0, 0, 0, 0, 0, 0, 0]  block_version=9.1.01
  Mux : xbsIndex_r4/Mux  inputs=2  en=off  latency=1  precision=Full  arith_type="Signed  (2's comp)"  n_bits=8  bin_pt=2  quantization=Truncate  overflow=Wrap  dbl_ovrd=off  block_type=mux
      settings: xl_area=[0, 0, 0, 0, 0, 0, 0]  block_version=9.1.01
  Relational : xbsIndex_r4/Relational  mode=a<b  en=off  latency=0  dbl_ovrd=off  block_type=relational
      settings: xl_area=[0, 0, 0, 0, 0, 0, 0]  block_version=9.1.01
  delay : Subsystem  AncestorBlock=casper_library/Delays/delay_bram  mask(delay_bram){DelayLen=acc_len, bram_latency=bram_latency}
      mask prompts: DelayLen "Delay By:"; bram_latency "BRAM Latency"
      mask help: A delay block that uses BRAM for its storage.
      mask init:
      | if (DelayLen <= bram_latency)
      | 	error('delay value must be greater than BRAM Latency');
      | end
      | BitWidth = max(ceil(log2(DelayLen)), 2);
      mask Help: eval('xlWeb([getenv(''MLIB_ROOT''), ''\doc\html\sp_delay_bram\sp_delay_bram.html''])')
  dual_pol_cmac : Subsystem
  a_del_out : Outport  OutDataType=sfix(16)  OutScaling=2^0
  a_ndel_out : Outport  Port=2  OutDataType=sfix(16)  OutScaling=2^0
  a_end_out : Outport  Port=3  OutDataType=sfix(16)  OutScaling=2^0
  acc_out : Outport  Port=4  OutDataType=sfix(16)  OutScaling=2^0
  valid_out : Outport  Port=5  OutDataType=sfix(16)  OutScaling=2^0
  rst_out : Outport  Port=6  OutDataType=sfix(16)  OutScaling=2^0
  sync_out : Outport  Port=7  OutDataType=sfix(16)  OutScaling=2^0
  wires:
  delay/1(Out1) -> Delay3/1
  Mux/1 -> dual_pol_cmac/2(a2)
  Counter/1 -> Relational/1
  Constant/1 -> Relational/2
  Relational/1 -> Convert/1
  Convert/1 -> Mux/1
  rst/1 -> Delay1/1, Counter/1
  a_del/1 -> delay/1(In1)
  dual_pol_cmac/1(acc_out) -> acc_out/1
  acc_in/1 -> dual_pol_cmac/3(acc_in)
  dual_pol_cmac/2(valid_out) -> valid_out/1
  valid_in/1 -> dual_pol_cmac/5(valid_in)
  a_ndel/1 -> Mux/2, Delay7/1
  a_end/1 -> Mux/3, Delay8/1
  Delay3/1 -> dual_pol_cmac/1(a1), a_del_out/1
  Delay7/1 -> a_ndel_out/1
  Delay8/1 -> a_end_out/1
  Delay1/1 -> dual_pol_cmac/4(sync), rst_out/1
  sync1/1 -> sync_out/1

== system test_xeng_2/xeng_static/baseline_tap4 ==
  a_del : Inport  OutDataType=sfix(16)  OutScaling=2^0
  a_ndel : Inport  Port=2  OutDataType=sfix(16)  OutScaling=2^0
  a_end : Inport  Port=3  OutDataType=sfix(16)  OutScaling=2^0
  acc_in : Inport  Port=4  OutDataType=sfix(16)  OutScaling=2^0
  valid_in : Inport  Port=5  OutDataType=sfix(16)  OutScaling=2^0
  rst : Inport  Port=6  OutDataType=sfix(16)  OutScaling=2^0
  sync1 : Inport  Port=7  OutDataType=sfix(16)  OutScaling=2^0
  Constant : xbsIndex_r4/Constant  arith_type=Unsigned  const=ant_sep * acc_len  n_bits=ant_bits + bit_growth  bin_pt=0  explicit_period=off  period=1  equ=P=C  opselect=C  inp2=PCIN>>17  opr=+  inp1=P  carry=CIN  dbl_ovrd=off  block_type=constant
      settings: block_version=9.1.01
  Convert : xbsIndex_r4/Convert  arith_type=Unsigned  n_bits=1  bin_pt=0  quantization=Truncate  overflow=Wrap  latency=0  dbl_ovrd=off  pipeline=off  block_type=convert
      settings: xl_area=[0, 0, 0, 0, 0, 0, 0]
  Counter : xbsIndex_r4/Counter  cnt_type=Count Limited  cnt_to=n_ants * acc_len - 1  operation=Up  start_count=0  cnt_by_val=1  arith_type=Unsigned  n_bits=ant_bits + bit_growth  bin_pt=0  load_pin=off  rst=on  en=off  explicit_period=off  period=1  dbl_ovrd=off  use_behavioral_HDL=off  use_rpm=on  implementation=Fabric  block_type=counter
      settings: xl_area=[0, 0, 0, 0, 0, 0, 0]  block_version=9.1.01
  Delay{1,3,7..8} (4 alike) : xbsIndex_r4/Delay  en=off  latency=1  dbl_ovrd=off  reg_retiming=off  block_type=delay
      settings: xl_area=[0, 0, 0, 0, 0, 0, 0]  block_version=9.1.01
  Mux : xbsIndex_r4/Mux  inputs=2  en=off  latency=1  precision=Full  arith_type="Signed  (2's comp)"  n_bits=8  bin_pt=2  quantization=Truncate  overflow=Wrap  dbl_ovrd=off  block_type=mux
      settings: xl_area=[0, 0, 0, 0, 0, 0, 0]  block_version=9.1.01
  Relational : xbsIndex_r4/Relational  mode=a<b  en=off  latency=0  dbl_ovrd=off  block_type=relational
      settings: xl_area=[0, 0, 0, 0, 0, 0, 0]  block_version=9.1.01
  delay : Subsystem  AncestorBlock=casper_library/Delays/delay_bram  mask(delay_bram){DelayLen=acc_len, bram_latency=bram_latency}
      mask prompts: DelayLen "Delay By:"; bram_latency "BRAM Latency"
      mask help: A delay block that uses BRAM for its storage.
      mask init:
      | if (DelayLen <= bram_latency)
      | 	error('delay value must be greater than BRAM Latency');
      | end
      | BitWidth = max(ceil(log2(DelayLen)), 2);
      mask Help: eval('xlWeb([getenv(''MLIB_ROOT''), ''\doc\html\sp_delay_bram\sp_delay_bram.html''])')
  dual_pol_cmac : Subsystem
  a_del_out : Outport  OutDataType=sfix(16)  OutScaling=2^0
  a_ndel_out : Outport  Port=2  OutDataType=sfix(16)  OutScaling=2^0
  a_end_out : Outport  Port=3  OutDataType=sfix(16)  OutScaling=2^0
  acc_out : Outport  Port=4  OutDataType=sfix(16)  OutScaling=2^0
  valid_out : Outport  Port=5  OutDataType=sfix(16)  OutScaling=2^0
  rst_out : Outport  Port=6  OutDataType=sfix(16)  OutScaling=2^0
  sync_out : Outport  Port=7  OutDataType=sfix(16)  OutScaling=2^0
  wires:
  delay/1(Out1) -> Delay3/1
  Mux/1 -> dual_pol_cmac/2(a2)
  Counter/1 -> Relational/1
  Constant/1 -> Relational/2
  Relational/1 -> Convert/1
  Convert/1 -> Mux/1
  rst/1 -> Delay1/1, Counter/1
  a_del/1 -> delay/1(In1)
  dual_pol_cmac/1(acc_out) -> acc_out/1
  acc_in/1 -> dual_pol_cmac/3(acc_in)
  dual_pol_cmac/2(valid_out) -> valid_out/1
  valid_in/1 -> dual_pol_cmac/5(valid_in)
  a_ndel/1 -> Mux/2, Delay7/1
  a_end/1 -> Mux/3, Delay8/1
  Delay3/1 -> dual_pol_cmac/1(a1), a_del_out/1
  Delay7/1 -> a_ndel_out/1
  Delay8/1 -> a_end_out/1
  Delay1/1 -> dual_pol_cmac/4(sync), rst_out/1
  sync1/1 -> sync_out/1
